simulink subsystem "CheckPWParam"  (R2023b)
settings: Solver=VariableStepAuto  StartTime=0.0  StopTime=10.0  RelTol=1e-3
libraries: simulink x1
settings Model: Creator=dfurodet  LastModifiedBy=dfurodet

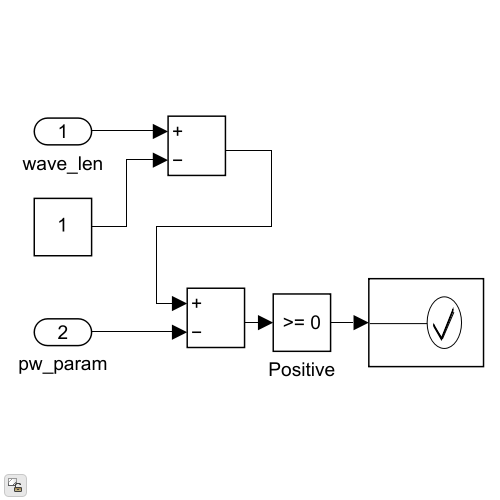
[thumbnail: Simulink's stored preview of the top-level diagram]
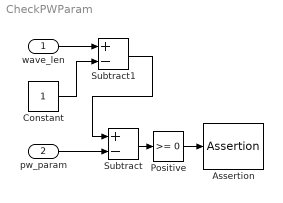
== system CheckPWParam ==
  wave_len : Inport
  pw_param : Inport  Port=2
  Assertion : Assertion
  Constant : Constant
  Positive : simulink/Logic and Bit Operations/Compare To Zero  relop=>=  OutDataTypeStr=boolean
  Subtract : Sum  Inputs=+-
  Subtract1 : Sum  Inputs=+-
  wires:
  wave_len/1 -> Subtract1/1
  Positive/1 -> Assertion/1
  Subtract/1 -> Positive/1
  pw_param/1 -> Subtract/2
  Constant/1 -> Subtract1/2
  Subtract1/1 -> Subtract/1
